simulink model "rete_digitale_duale"  (R2017a)
settings: Solver=VariableStepAuto  StartTime=0.0  StopTime=10.0  RelTol=1e-3
values from neighbouring files (symbols this model uses):
  beta0 = b0    (= 0)    [SistemaDigitaleInAvanti.m]    (also in SistemaDigitaleIndietro.m = 0.000499749875187)
  beta1 = -2*b0 + b1*Tc    (= 0)    [SistemaDigitaleInAvanti.m]    (also in SistemaDigitaleIndietro.m)
  beta2 = b0 - b1*Tc + b2*Tc^2    (= 0.001)    [SistemaDigitaleInAvanti.m]    (also in SistemaDigitaleIndietro.m = 0)
undefined symbols (not defined in the file or in its folder): alpha1, alpha2
settings Model: Creator=Enrico Donato  LastModifiedBy=Enrico Donato

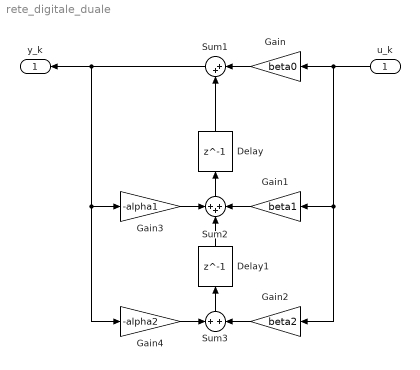
== system rete_digitale_duale ==
  u_k : Inport
  Delay : Delay  DelayLength=1  InitialCondition=0
  Delay1 : Delay  DelayLength=1  InitialCondition=0
  Gain : Gain  Gain=beta0
  Gain1 : Gain  Gain=beta1
  Gain2 : Gain  Gain=beta2
  Gain3 : Gain  Gain=-alpha1
  Gain4 : Gain  Gain=-alpha2
  Sum1 : Sum  Inputs=|++
  Sum2 : Sum  Inputs=+++
  Sum3 : Sum
  y_k : Outport
  wires:
  Gain3/1 -> Sum2/1
  Gain1/1 -> Sum2/3
  Delay1/1 -> Sum2/2
  Sum2/1 -> Delay/1
  Gain4/1 -> Sum3/1
  Sum3/1 -> Delay1/1
  Gain2/1 -> Sum3/2
  Gain/1 -> Sum1/1
  Delay/1 -> Sum1/2
  u_k/1 -> Gain2/1, Gain1/1, Gain/1
  Sum1/1 -> Gain4/1, Gain3/1, y_k/1
